simulink library "quadLibrary"  (R2015b)
settings: Solver=VariableStepAuto  StartTime=0.0  StopTime=10.0  RelTol=1e-3
libraries: simulink x1
settings Model: Creator=Nik Descher  LastModifiedBy=Nik Descher

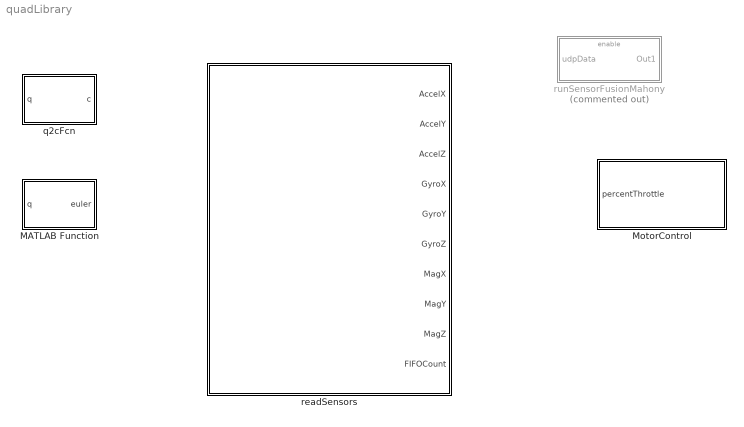
== system quadLibrary ==
  MATLAB Function : MATLAB Function  TreatAsAtomicUnit=on
  MotorControl : Subsystem  TreatAsAtomicUnit=on
      settings: RTWSystemCode=Inline  RTWFcnNameOpts=Use subsystem name  RTWFileNameOpts=Use subsystem name
  q2cFcn : MATLAB Function  TreatAsAtomicUnit=on
  readSensors : Subsystem  TreatAsAtomicUnit=on  SystemSampleTime=1/1000
  runSensorFusionMahony : Subsystem  Commented=on  TreatAsAtomicUnit=on

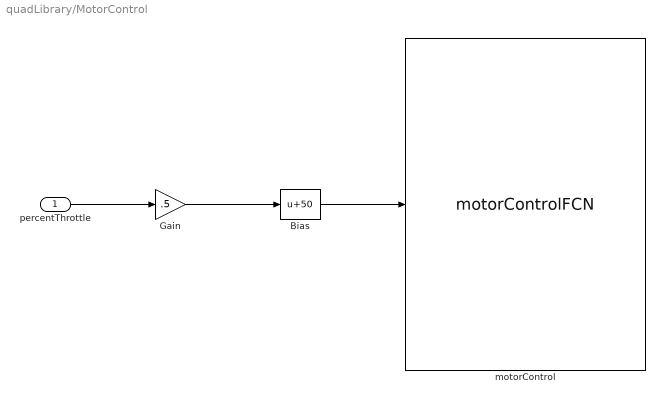
== system quadLibrary/MotorControl ==
  percentThrottle : Inport  OutMin=0  OutMax=100  OutDataTypeStr=single  PortDimensions=4  SampleTime=1/50
  Bias : Bias  Bias=50
  Gain : Gain  Gain=.5
  motorControl : S-Function  InitFcn=try, set_param(gcb,'FunctionName','motorControlFCN'), end  FunctionName=motorControlFCN  SFunctionModules=motorControlFCN_wrapper  SFunctionDeploymentMode=off  EnableBusSupport=off  mask(S-Function Builder){Parameter1=0, Parameter2=0}
      mask prompts: Parameter1 "High Reg Address"; Parameter2 "Low Reg Address"
      mask help: Simulink:masks:SFunctionBuilder_MD
      mask init:
      | val = [[.9  0.75 0.75 1 1 .9 .9 1]',[1 1 0.75 0.75 .9 .9 1 .9]'];try , sys = get_param(gcb,'SfunBuilderFcnName');if isempty(sys), sys = get_param(gcb,'FunctionName'); end,catch, sys = get_param(gcb,'FunctionName'); end
      settings: CopyFcn=set_param(gcbh,'LinkStatus','none')  PreSaveFcn=try, set_param(gcb,'FunctionName','motorControlFCN'), end  OpenFcn=sfunctionwizard(gcbh)
      mask Display: plot(val(:,1),val(:,2)),disp(sys), port_label('input',1,'motorSpeed')
  wires:
  Bias/1 -> motorControl/1
  percentThrottle/1 -> Gain/1
  Gain/1 -> Bias/1

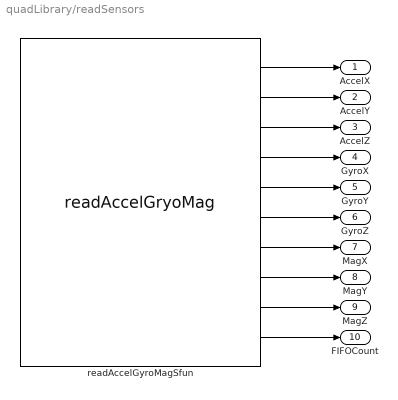
== system quadLibrary/readSensors ==
  readAccelGyroMagSfun : S-Function  InitFcn=try, set_param(gcb,'FunctionName','readAccelGryoMag'), end  FunctionName=readAccelGryoMag  SFunctionModules=readAccelGryoMag_wrapper  SFunctionDeploymentMode=off  EnableBusSupport=off  mask(S-Function Builder){Parameter1=0, Parameter2=0}
      mask prompts: Parameter1 "High Reg Address"; Parameter2 "Low Reg Address"
      mask help: Simulink:masks:SFunctionBuilder_MD
      mask init: same as quadLibrary/MotorControl/motorControl
      settings: CopyFcn=set_param(gcbh,'LinkStatus','none')  PreSaveFcn=try, set_param(gcb,'FunctionName','readAccelGryoMag'), end  OpenFcn=sfunctionwizard(gcbh)
      mask Display: plot(val(:,1),val(:,2)),disp(sys), port_label('output',1,'AccelX'), port_label('output',2,'AccelY'), port_label('output',3,'AccelZ'), port_label('output',4,'GyroX'), port_label('output',5,'GyroY'), port_label('output',6,'GyroZ'), port_label('output',7,'MagX'), port_label('output',8,'MagY'), port_label('output',9,'MagZ'), port_label('output',10,'FIFOCount')
  AccelX : Outport
  AccelY : Outport  Port=2
  AccelZ : Outport  Port=3
  GyroX : Outport  Port=4
  GyroY : Outport  Port=5
  GyroZ : Outport  Port=6
  MagX : Outport  Port=7
  MagY : Outport  Port=8
  MagZ : Outport  Port=9
  FIFOCount : Outport  Port=10
  wires:
  readAccelGyroMagSfun/10 -> FIFOCount/1
  readAccelGyroMagSfun/5 -> GyroY/1
  readAccelGyroMagSfun/2 -> AccelY/1
  readAccelGyroMagSfun/1 -> AccelX/1
  readAccelGyroMagSfun/4 -> GyroX/1
  readAccelGyroMagSfun/6 -> GyroZ/1
  readAccelGyroMagSfun/7 -> MagX/1
  readAccelGyroMagSfun/3 -> AccelZ/1
  readAccelGyroMagSfun/9 -> MagZ/1
  readAccelGyroMagSfun/8 -> MagY/1

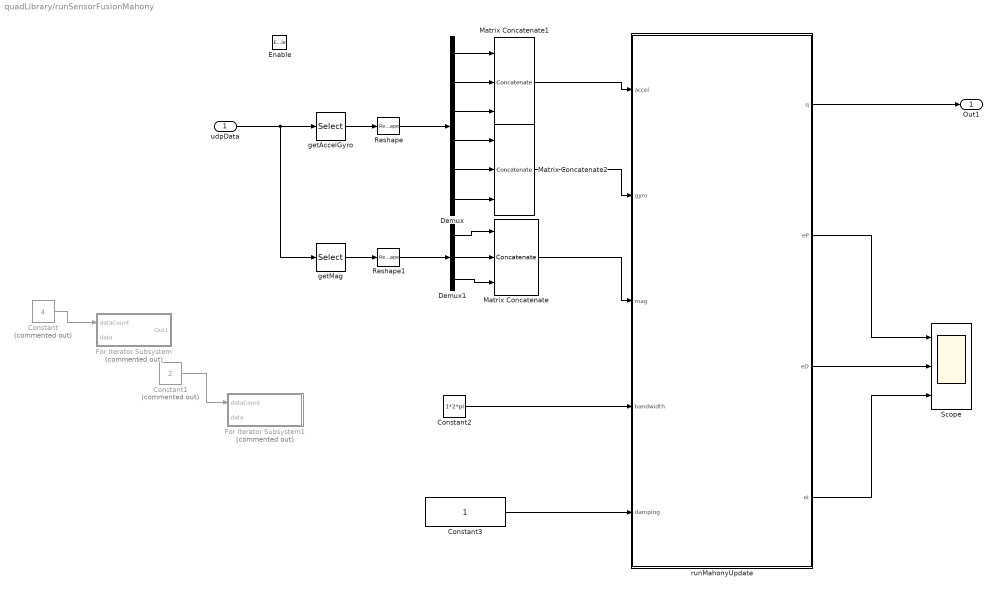
== system quadLibrary/runSensorFusionMahony ==
  udpData : Inport
  Enable : EnablePort
  Constant : Constant  Commented=on  Value=4
  Constant1 : Constant  Commented=on  Value=2
  Constant2 : Constant  Value=1*2*pi  OutDataTypeStr=single
  Constant3 : Constant  OutDataTypeStr=single
  Demux : Demux  Outputs=6
  Demux1 : Demux  Outputs=3
  For Iterator Subsystem : Subsystem  Commented=on  TreatAsAtomicUnit=on
  For Iterator Subsystem1 : Subsystem  Commented=on  TreatAsAtomicUnit=on
  Matrix Concatenate : Concatenate  NumInputs=3  Mode=Multidimensional array
  Matrix Concatenate1 : Concatenate  NumInputs=3  Mode=Multidimensional array
  Matrix Concatenate2 : Concatenate  NumInputs=3  Mode=Multidimensional array
  Reshape : Reshape
  Reshape1 : Reshape
  Scope : Scope  NumInputPorts=3
  getAccelGyro : Selector  InputPortWidth=31  IndexOptions=Index vector (dialog)  Indices=1:24  OutputSizes=1
  getMag : Selector  InputPortWidth=31  IndexOptions=Index vector (dialog)  Indices=25:30  OutputSizes=1
  runMahonyUpdate : MATLAB Function  TreatAsAtomicUnit=on
  Out1 : Outport
  wires:
  runMahonyUpdate/4(eI) -> Scope/3
  runMahonyUpdate/3(eD) -> Scope/2
  runMahonyUpdate/2(eP) -> Scope/1
  runMahonyUpdate/1(q) -> Out1/1
  Constant3/1 -> runMahonyUpdate/5(damping)
  Constant2/1 -> runMahonyUpdate/4(bandwidth)
  Matrix Concatenate/1 -> runMahonyUpdate/3(mag)
  Matrix Concatenate2/1 -> runMahonyUpdate/2(gyro)
  Matrix Concatenate1/1 -> runMahonyUpdate/1(accel)
  Demux/6 -> Matrix Concatenate2/3
  Demux/5 -> Matrix Concatenate2/2
  Demux/4 -> Matrix Concatenate2/1
  Demux/1 -> Matrix Concatenate1/1
  Demux/3 -> Matrix Concatenate1/3
  Demux/2 -> Matrix Concatenate1/2
  Demux1/3 -> Matrix Concatenate/3
  Demux1/1 -> Matrix Concatenate/1
  Demux1/2 -> Matrix Concatenate/2
  getMag/1 -> Reshape1/1
  udpData/1 -> getAccelGyro/1, getMag/1
  Reshape1/1 -> Demux1/1
  Reshape/1 -> Demux/1
  getAccelGyro/1 -> Reshape/1
  Constant1/1 -> For Iterator Subsystem1/1(dataCount)
  Constant/1 -> For Iterator Subsystem/1(dataCount)

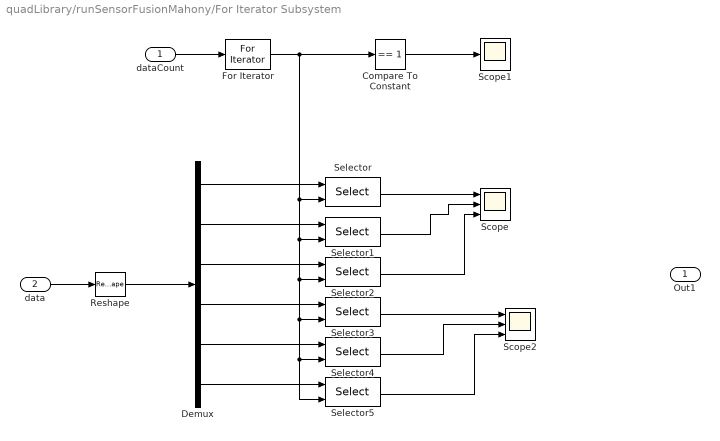
== system quadLibrary/runSensorFusionMahony/For Iterator Subsystem ==
  dataCount : Inport
  data : Inport  Port=2
  Compare To Constant : simulink/Logic and Bit Operations/Compare To Constant  relop===  const=1  OutDataTypeStr=boolean
  Demux : Demux  Outputs=6
  For Iterator : ForIterator  IterationSource=external
  Reshape : Reshape
  Scope : Scope  NumInputPorts=3
  Scope1 : Scope
  Scope2 : Scope  NumInputPorts=3
  Selector{,1..5} (6 alike) : Selector  InputPortWidth=4  IndexOptions=Index vector (port)  Indices=[1 3]  OutputSizes=1
  Out1 : Outport
  wires:
  Selector5/1 -> Scope2/3
  Selector4/1 -> Scope2/2
  Selector3/1 -> Scope2/1
  Reshape/1 -> Demux/1
  Compare To Constant/1 -> Scope1/1
  Selector2/1 -> Scope/3
  Selector1/1 -> Scope/2
  Selector/1 -> Scope/1
  Demux/6 -> Selector5/1
  Demux/5 -> Selector4/1
  Demux/4 -> Selector3/1
  Demux/3 -> Selector2/1
  Demux/2 -> Selector1/1
  For Iterator/1 -> Selector/2, Selector1/2, Selector2/2, Selector3/2, Selector4/2, Selector5/2, Compare To Constant/1
  Demux/1 -> Selector/1
  data/1 -> Reshape/1
  dataCount/1 -> For Iterator/1

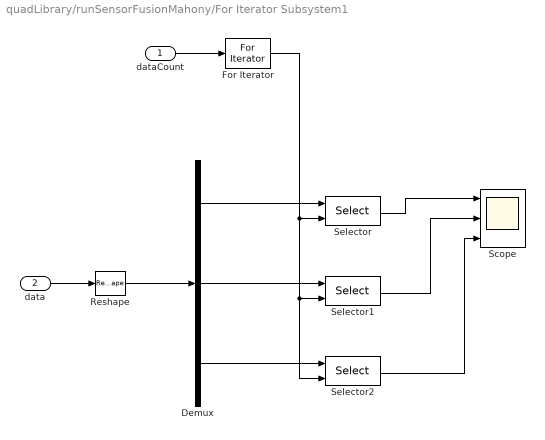
== system quadLibrary/runSensorFusionMahony/For Iterator Subsystem1 ==
  dataCount : Inport
  data : Inport  Port=2
  Demux : Demux  Outputs=3
  For Iterator : ForIterator  IterationSource=external
  Reshape : Reshape
  Scope : Scope  NumInputPorts=3
  Selector : Selector  InputPortWidth=2  IndexOptions=Index vector (port)  Indices=[1 3]  OutputSizes=1
  Selector1 : Selector  InputPortWidth=2  IndexOptions=Index vector (port)  Indices=[1 3]  OutputSizes=1
  Selector2 : Selector  InputPortWidth=2  IndexOptions=Index vector (port)  Indices=[1 3]  OutputSizes=1
  wires:
  dataCount/1 -> For Iterator/1
  data/1 -> Reshape/1
  Demux/1 -> Selector/1
  For Iterator/1 -> Selector2/2, Selector1/2, Selector/2
  Demux/2 -> Selector1/1
  Demux/3 -> Selector2/1
  Selector/1 -> Scope/1
  Selector1/1 -> Scope/2
  Selector2/1 -> Scope/3
  Reshape/1 -> Demux/1

== matlab function quadLibrary/runSensorFusionMahony/runMahonyUpdate ==
  data: accel input single size=[3 4]; q output; gyro input single size=[3 4]; mag input single size=[3 2]; bandwidth input; damping input; eP output; eD output; eI output
function [q,eP,eD,eI] = runMahonyUpdate(accel,gyro,mag,bandwidth,damping)
persistent qLocal
if isempty(qLocal)
    qLocal=single([ 1 0 0 0]);
end

magInterp=interp1([1 4],mag',[1 2 3 4],'linear')';

for i=1:4
    [qLocal,eP,eD,eI]=UpdateMahony(qLocal,gyro(:,i),accel(:,i),magInterp(:,i),bandwidth,damping);
end

q=qLocal;



 function [q,eP,eD,eI] = UpdateMahony(q,Gyroscope, Accelerometer, Magnetometer,bandwidth,damping)
     persistent eInt eLast
     if isempty(eInt)
         eInt=single([0; 0; 0]);
     end
     if abs(bandwidth)<1e-4 && abs(damping)<1e-4
         q=single([1 0 0 0]);
         eP=single([0;0;0]);
         eD=eP;
         eI=eP;
         return;
     end
%      bandwidth = (1*2*pi);
%      damping=1;
     Ki=bandwidth^2*bandwidth;
     Kp=bandwidth^2+2*damping*bandwidth*bandwidth;
     Kd=2*damping*bandwidth+bandwidth;
% 
%      Ki=0;
%      Kp=1;
%      Kd=0;
     
     SamplePeriod=5/1000;
     % Normalise accelerometer measurement
%      if(norm(Accelerometer) == 0), return; end   % handle NaN
     Accelerometer = Accelerometer / norm(Accelerometer);    % normalise magnitude
     
     % Normalise magnetometer measurement
%      if(norm(Magnetometer) == 0), return; end    % handle NaN
     Magnetometer = Magnetometer / norm(Magnetometer);   % normalise magnitude
     
     % Reference direction of Earth's magnetic feild
     h = quaternProd(q, quaternProd([0; Magnetometer], quaternConj(q)));
     b = [0; norm([h(2); h(3)]); 0; h(4)];
     
     % Estimated direction of gravity and magnetic field
     v = [2*(q(2)*q(4) - q(1)*q(3))
         2*(q(1)*q(2) + q(3)*q(4))
         q(1)^2 - q(2)^2 - q(3)^2 + q(4)^2];
     w = [2*b(2)*(0.5 - q(3)^2 - q(4)^2) + 2*b(4)*(q(2)*q(4) - q(1)*q(3))
         2*b(2)*(q(2)*q(3) - q(1)*q(4)) + 2*b(4)*(q(1)*q(2) + q(3)*q(4))
         2*b(2)*(q(1)*q(3) + q(2)*q(4)) + 2*b(4)*(0.5 - q(2)^2 - q(3)^2)];
     
     % Error is sum of cross product between estimated direction and measured direction of fields
     e = cross(Accelerometer, v) + cross(Magnetometer, w);
     if(Ki > 0)
         eInt = eInt + e * SamplePeriod;
     else
         eInt = single([0; 0; 0]);
     end
     if isempty(eLast)
         eLast=e;
     end
     
     % Apply feedback terms
     eP=e;
     eD=e-eLast;
     eI=eInt;
     Gyroscope = Gyroscope + Kp * eP + Ki * eInt + Kd * (eD) / SamplePeriod;
     eLast=e;
     
     % Compute rate of change of quaternion
     qDot = 0.5 * quaternProd(q, [0 Gyroscope(1) Gyroscope(2) Gyroscope(3)]);
     
     % Integrate to yield quaternion
     q = q + qDot * SamplePeriod;
     q = q / norm(q); % normalise quaternion
     

function ab = quaternProd(a, b)
    ab=zeros(1,4);
%QUATERNPROD Calculates the quaternion product
%
%   ab = quaternProd(a, b)
%
%   Calculates the quaternion product of quaternion a and b.
%
%   For more information see:
%   http://www.x-io.co.uk/node/8#quaternions
%
%	Date          Author          Notes
%	27/09/2011    SOH Madgwick    Initial release

    ab(1) = a(1).*b(1)-a(2).*b(2)-a(3).*b(3)-a(4).*b(4);
    ab(2) = a(1).*b(2)+a(2).*b(1)+a(3).*b(4)-a(4).*b(3);
    ab(3) = a(1).*b(3)-a(2).*b(4)+a(3).*b(1)+a(4).*b(2);
    ab(4) = a(1).*b(4)+a(2).*b(3)-a(3).*b(2)+a(4).*b(1);

function qConj = quaternConj(q)
%QUATERN2ROTMAT Converts a quaternion to its conjugate
%
%   qConj = quaternConj(q)
%
%   Converts a quaternion to its conjugate.
%
%   For more information see:
%   http://www.x-io.co.uk/node/8#quaternions
%
%	Date          Author          Notes
%	27/09/2011    SOH Madgwick    Initial release

    qConj = [q(1) -q(2) -q(3) -q(4)];

== matlab function quadLibrary/MATLAB Function ==
  data: q input single size=4; euler output single size=[1 3]
function euler = quatern2euler(q)
%#codegen

%QUATERN2EULER Converts a quaternion orientation to ZYX Euler angles
%
%   q = quatern2euler(q)
%
%   Converts a quaternion orientation to ZYX Euler angles where phi is a
%   rotation around X, theta around Y and psi around Z.
%
%   For more information see:
%   http://www.x-io.co.uk/node/8#quaternions
%
%	Date          Author          Notes
%	27/09/2011    SOH Madgwick    Initial release
R=zeros(3,'single');
    R(1,1) = 2.*q(1).^2-1+2.*q(2).^2;
    R(2,1) = 2.*(q(2).*q(3)-q(1).*q(4));
    R(3,1) = 2.*(q(2).*q(4)+q(1).*q(3));
    R(3,2) = 2.*(q(3).*q(4)-q(1).*q(2));
    R(3,3) = 2.*q(1).^2-1+2.*q(4).^2;

    phi = atan2(R(3,2), R(3,3) );
    theta = -atan(R(3,1) ./ sqrt(1-R(3,1).^2) );
    psi = atan2(R(2,1), R(1,1) );

    euler = [phi(1)' theta(1)' psi(1)'];
end

== matlab function quadLibrary/q2cFcn ==
  data: q input single size=[4 1]; c output single size=[3 3]
function c=q2c(q)
%#codegen
% Q2C computes a transformation matrix (c) from the given
% quaternion (q).
%
%  usage: c=q2c(q)
%
% Transformation matrix is of the form:
%
%     C = Cbn
%     q = qnb
%
%     where q(1)   = scalar part
%           q(2-4) = vector part
%
%    Vb = C * Vn
%    Ib = C'* In * C
%
q0=q(1); % scalar part
q1=q(2);
q2=q(3);
q3=q(4);
%
q1q2=q1*q2;
q1q3=q1*q3;
q1q0=q1*q0;
q2q3=q2*q3;
q2q0=q2*q0;
q3q0=q3*q0;
q1q1=q1*q1;
q2q2=q2*q2;
q3q3=q3*q3;
%
c=single(zeros(3,3));
s1=single(1.0);
s2=single(2.0);

c(1,1)=s1-s2*(q2q2+q3q3);
c(1,2)=s2*(q1q2+q3q0);
c(1,3)=s2*(q1q3-q2q0);
c(2,1)=s2*(q1q2-q3q0);
c(2,2)=s1-s2*(q1q1+q3q3);
c(2,3)=s2*(q2q3+q1q0);
c(3,1)=s2*(q1q3+q2q0);
c(3,2)=s2*(q2q3-q1q0);
c(3,3)=s1-s2*(q1q1+q2q2);
